simulink model "powerLoad"  (R2019b)
settings: Solver=VariableStepAuto  StartTime=0.0  StopTime=500  RelTol=1e-3
InitFcn:
  | Rho_air= 1.225;
  | C_d=0.9;
  | A_d= 0.4;
  | Static_Friction_Coefficient =0.0015;
  | Dynamic_Friction_Coefficient= 0.0015;
  | Cyclist_weight=85;
  | Vehicle_mass = 25;
  | Trailer_mass = 50;
  | g = 9.81;
  | Wheel_mass = 0.25;
  | Tire_mass = 0.25;
  | Abs = 1;
  | Bb=0.2;
  | Wheel_Radius = 0.3;
  | F_Rider = 70;
  | Wheel_Inertia=0.0225;
  | Braking_Pressure=100;
  | Crank_Length = 0.150;
  | Angle_of_crank = [0:1:360;0:1:360;]';
  | Number_of_brake_pad = 2;
  | Coefficient_of_Brake_friction = 0.9;
  | Effective_Radius_of_Disc = 0.16;
  | Outer_Radius_of_Brake = 0.18;
  | Inner_Radius_of_Brake = 0.14;
  | Disc_Mass=0;
  | Heat_capacity=0;
  | Surface_Temp=0;
  | Ambient_Temp=0;
  | Thermal_Conductivity=1;
  | 
  | Motor_torque_constant = 0.75; % NM/A
  | Kb = (51.7/(1000*2*pi/60)); %or  V/Wm (wm in rps) volt/rps
  | Jm =10.2 *10^-3; %kgm^2
  | Bm = ((Motor_torque_constant)*(17)/(1000*2*pi/60));
  | Motor_resistance =88*10^-2; %ohm
  | L = 0.36*10^-3;% H(henry)
  | alpha_Conductor =0.0040;
  | Ref_Temp = 25;
  | Alpha_Magnet = -0.0020;
  | 
  | Internal_Resistance =95*10^-3; %ohm
  | capacity =19.5 ; %Ah
  | SOC_initial = 100;
  | Polarization_Resistance = 95*10^-3;
  | Polarization_Capacitance = 1*10^-7;
undefined symbols (not defined in the file or in its folder): sigbuilder_block, V
libraries: simulink x2
(part 2 of 2)

== system powerLoad/Bike_Mechanics_subsystem/If Action Subsystem6 ==
  In1 : Inport
  Action Port : ActionPort  ActionPortLabel=else
  Gain : Gain
  Out1 : Outport
  wires:
  Gain/1 -> Out1/1
  In1/1 -> Gain/1

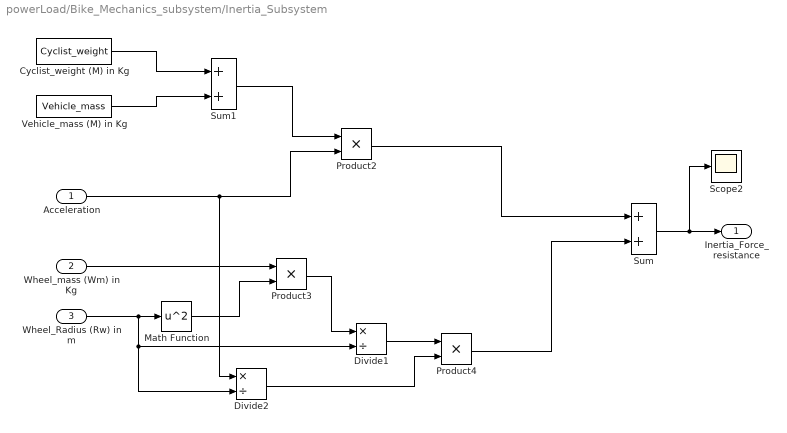
== system powerLoad/Bike_Mechanics_subsystem/Inertia_Subsystem ==
  Acceleration : Inport
  Wheel_mass (Wm) in Kg : Inport  Port=2
  Wheel_Radius (Rw) in m : Inport  Port=3
  Cyclist_weight (M) in Kg : Constant  Value=Cyclist_weight  SampleTime=-1
  Divide1 : Product  Inputs=*/
  Divide2 : Product  Inputs=*/
  Math Function : Math  Operator=square  SaturateOnIntegerOverflow=on
  Product2 : Product
  Product3 : Product
  Product4 : Product
  Scope2 : Scope
  Sum : Sum
  Sum1 : Sum
  Vehicle_mass (M) in Kg : Constant  Value=Vehicle_mass  SampleTime=-1
  Inertia_Force_resistance : Outport
  wires:
  Wheel_Radius (Rw) in m/1 -> Divide2/2, Divide1/2, Math Function/1
  Wheel_mass (Wm) in Kg/1 -> Product3/1
  Math Function/1 -> Product3/2
  Cyclist_weight (M) in Kg/1 -> Sum1/1
  Vehicle_mass (M) in Kg/1 -> Sum1/2
  Acceleration/1 -> Divide2/1, Product2/2
  Sum1/1 -> Product2/1
  Product3/1 -> Divide1/1
  Divide1/1 -> Product4/1
  Divide2/1 -> Product4/2
  Sum/1 -> Scope2/1, Inertia_Force_resistance/1
  Product2/1 -> Sum/1
  Product4/1 -> Sum/2

== system powerLoad/Bike_Mechanics_subsystem/Inertia_Subsystem1 ==
  Acceleration : Inport
  Gain : Gain
  Product2 : Product
  Scope2 : Scope
  Vehicle_mass (M) in Kg : Constant  Value=Trailer_mass  SampleTime=-1
  Trailer_force : Outport
  wires:
  Product2/1 -> Gain/1
  Vehicle_mass (M) in Kg/1 -> Product2/1
  Acceleration/1 -> Product2/2
  Gain/1 -> Scope2/1, Trailer_force/1

== system powerLoad/Bike_Mechanics_subsystem/Pedallic_torque_subsystem ==
  Torque : Inport
  Gear_ratio : Inport  Port=2
  Divide : Product  Inputs=*/
  Divide1 : Product  Inputs=*/
  Scope : Scope
  Scope1 : Scope
  Scope2 : Scope
  "Wheel_radius (Rw) " : Constant  Value=Wheel_Radius  SampleTime=-1
  Drive_Force : Outport  VectorParamsAs1DForOutWhenUnconnected=off
  wires:
  Gear_ratio/1 -> Divide1/2
  Divide1/1 -> Scope/1, Divide/1
  "Wheel_radius (Rw) "/1 -> Divide/2
  Divide/1 -> Scope2/1, Drive_Force/1
  Torque/1 -> Divide1/1, Scope1/1

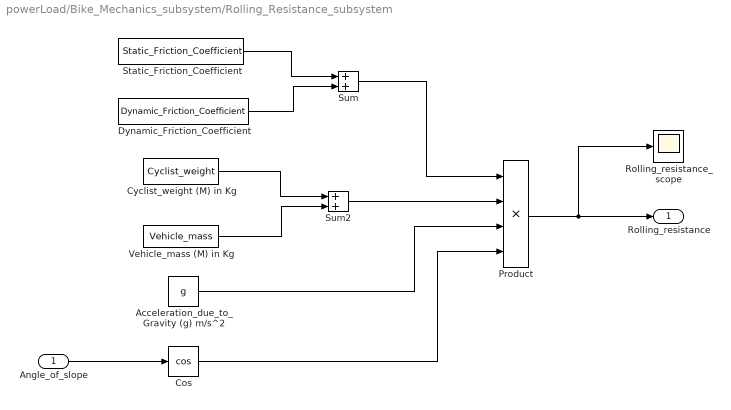
== system powerLoad/Bike_Mechanics_subsystem/Rolling_Resistance_subsystem ==
  Angle_of_slope : Inport
  Acceleration_due_to_Gravity (g) m/s^2 : Constant  Value=g  SampleTime=-1
  Cos : Trigonometry  Operator=cos
  Cyclist_weight (M) in Kg : Constant  Value=Cyclist_weight  SampleTime=-1
  Dynamic_Friction_Coefficient : Constant  Value=Dynamic_Friction_Coefficient  SampleTime=-1
  Product : Product  Inputs=4
  Rolling_resistance_scope : Scope
  Static_Friction_Coefficient : Constant  Value=Static_Friction_Coefficient  SampleTime=-1
  Sum : Sum  Inputs=+|+
  Sum2 : Sum
  Vehicle_mass (M) in Kg : Constant  Value=Vehicle_mass  SampleTime=-1
  Rolling_resistance : Outport  VectorParamsAs1DForOutWhenUnconnected=off
  wires:
  Acceleration_due_to_Gravity (g) m/s^2/1 -> Product/3
  Product/1 -> Rolling_resistance/1, Rolling_resistance_scope/1
  Cos/1 -> Product/4
  Angle_of_slope/1 -> Cos/1
  Static_Friction_Coefficient/1 -> Sum/1
  Dynamic_Friction_Coefficient/1 -> Sum/2
  Sum/1 -> Product/1
  Sum2/1 -> Product/2
  Cyclist_weight (M) in Kg/1 -> Sum2/1
  Vehicle_mass (M) in Kg/1 -> Sum2/2

== system powerLoad/Bike_Mechanics_subsystem/Subsystem2 ==
  Slope % : Inport
  Constant : Constant  Value=pi  SampleTime=-1
  Constant1 : Constant  Value=180
  Divide : Product  Inputs=*/
  Gain : Gain  Gain=1/1
  Product : Product
  Trigonometric Function : Trigonometry  Operator=atan
  alpha : Outport  VectorParamsAs1DForOutWhenUnconnected=off
  wires:
  Gain/1 -> Trigonometric Function/1
  Slope %/1 -> Gain/1
  Trigonometric Function/1 -> Product/1
  Product/1 -> alpha/1
  Constant/1 -> Divide/1
  Constant1/1 -> Divide/2
  Divide/1 -> Product/2

== system powerLoad/Controller/If Action Subsystem1 ==
  In1 : Inport
  Action Port : ActionPort  ActionPortLabel=if(u1<26)
  Gain : Gain
  Out1 : Outport
  wires:
  In1/1 -> Gain/1
  Gain/1 -> Out1/1

== system powerLoad/Controller/If Action Subsystem11 ==
  In1 : Inport
  Action Port : ActionPort  ActionPortLabel=if(u1 > 0)
  Gain : Gain  Gain=0
  Out1 : Outport
  wires:
  Gain/1 -> Out1/1
  In1/1 -> Gain/1

== system powerLoad/Controller/If Action Subsystem12 ==
  In1 : Inport
  Action Port : ActionPort  ActionPortLabel=else
  Gain : Gain
  Out1 : Outport
  wires:
  Gain/1 -> Out1/1
  In1/1 -> Gain/1

== system powerLoad/Controller/If Action Subsystem2 ==
  In1 : Inport
  Action Port : ActionPort  ActionPortLabel=if(u1 > 0)
  Gain : Gain  Gain=0
  Out1 : Outport
  wires:
  In1/1 -> Gain/1
  Gain/1 -> Out1/1

== system powerLoad/Controller/If Action Subsystem3 ==
  In1 : Inport
  Action Port : ActionPort  ActionPortLabel=else
  Gain : Gain
  Out1 : Outport
  wires:
  In1/1 -> Gain/1
  Gain/1 -> Out1/1

== system powerLoad/Controller/If Action Subsystem5 ==
  In1 : Inport
  Action Port : ActionPort  ActionPortLabel=if(u1 > 0)
  Gain : Gain  Gain=0
  Out1 : Outport
  wires:
  Gain/1 -> Out1/1
  In1/1 -> Gain/1

== system powerLoad/Controller/If Action Subsystem6 ==
  In1 : Inport
  Action Port : ActionPort  ActionPortLabel=else
  Gain : Gain
  Out1 : Outport
  wires:
  Gain/1 -> Out1/1
  In1/1 -> Gain/1

== system powerLoad/Controller/If Action Subsystem8 ==
  In1 : Inport
  Action Port : ActionPort  ActionPortLabel=else
  Gain : Gain  Gain=0
  Out1 : Outport
  wires:
  Gain/1 -> Out1/1
  In1/1 -> Gain/1

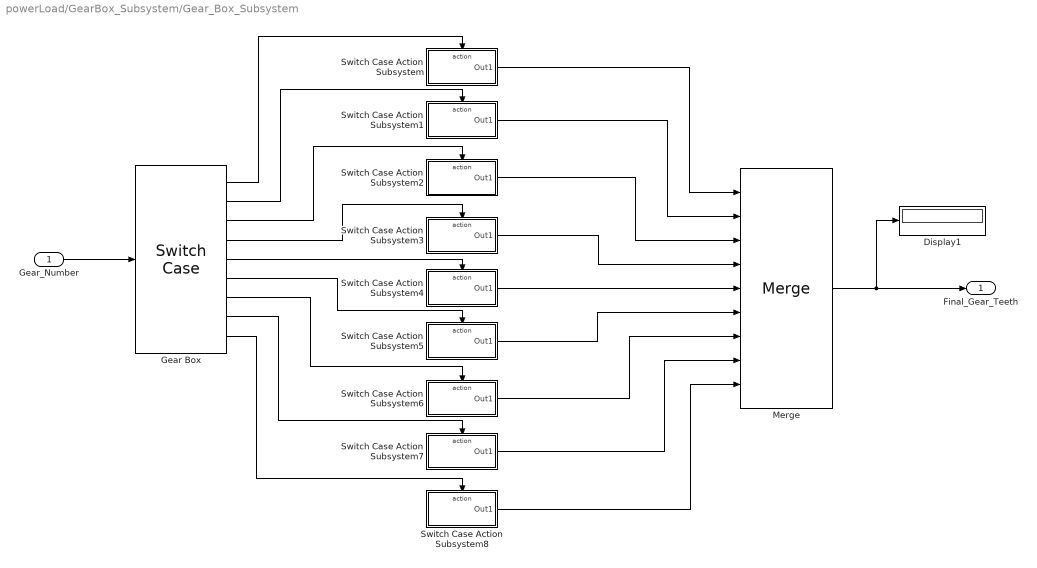
== system powerLoad/GearBox_Subsystem/Gear_Box_Subsystem ==
  Gear_Number : Inport
  Display1 : Display
  Gear Box : SwitchCase  CaseConditions={1,2,3,4,5,6,7,8,9}  ShowDefaultCase=off
  Merge : Merge  Inputs=9
  Switch Case Action Subsystem : Subsystem  TreatAsAtomicUnit=on
  Switch Case Action Subsystem1 : Subsystem  TreatAsAtomicUnit=on
  Switch Case Action Subsystem2 : Subsystem  TreatAsAtomicUnit=on
  Switch Case Action Subsystem3 : Subsystem  TreatAsAtomicUnit=on
  Switch Case Action Subsystem4 : Subsystem  TreatAsAtomicUnit=on
  Switch Case Action Subsystem5 : Subsystem  TreatAsAtomicUnit=on
  Switch Case Action Subsystem6 : Subsystem  TreatAsAtomicUnit=on
  Switch Case Action Subsystem7 : Subsystem  TreatAsAtomicUnit=on
  Switch Case Action Subsystem8 : Subsystem  TreatAsAtomicUnit=on
  Final_Gear_Teeth : Outport  VectorParamsAs1DForOutWhenUnconnected=off
  wires:
  Gear Box/5 -> Switch Case Action Subsystem4/Action
  Gear Box/2 -> Switch Case Action Subsystem1/Action
  Gear Box/4 -> Switch Case Action Subsystem3/Action
  Gear Box/9 -> Switch Case Action Subsystem8/Action
  Gear Box/7 -> Switch Case Action Subsystem6/Action
  Gear Box/6 -> Switch Case Action Subsystem5/Action
  Gear Box/3 -> Switch Case Action Subsystem2/Action
  Gear Box/1 -> Switch Case Action Subsystem/Action
  Merge/1 -> Display1/1, Final_Gear_Teeth/1
  Gear Box/8 -> Switch Case Action Subsystem7/Action
  Gear_Number/1 -> Gear Box/1
  Switch Case Action Subsystem8/1(Out1) -> Merge/9
  Switch Case Action Subsystem7/1(Out1) -> Merge/8
  Switch Case Action Subsystem6/1(Out1) -> Merge/7
  Switch Case Action Subsystem5/1(Out1) -> Merge/6
  Switch Case Action Subsystem4/1(Out1) -> Merge/5
  Switch Case Action Subsystem3/1(Out1) -> Merge/4
  Switch Case Action Subsystem2/1(Out1) -> Merge/3
  Switch Case Action Subsystem1/1(Out1) -> Merge/2
  Switch Case Action Subsystem/1(Out1) -> Merge/1

== system powerLoad/Motor_Subsystem/Magnetic_Flux_density_subsystem ==
  Ambient_temp_T : Inport
  Motor_torque_constant_at_Temp_T0 : Inport  Port=2
  Constant : Constant
  Product : Product
  Product1 : Product
  Reference_temp_T0 : Constant  Value=Ref_Temp
  Sum1 : Sum  Inputs=+-
  Sum2 : Sum
  Temperature_Coefficient : Constant  Value=Alpha_Magnet
  Motor_Torque_Constant_at_Temp_T : Outport  VectorParamsAs1DForOutWhenUnconnected=off
  wires:
  Motor_torque_constant_at_Temp_T0/1 -> Product1/1
  Product1/1 -> Motor_Torque_Constant_at_Temp_T/1
  Product/1 -> Sum2/2
  Constant/1 -> Sum2/1
  Sum2/1 -> Product1/2
  Temperature_Coefficient/1 -> Product/1
  Ambient_temp_T/1 -> Sum1/1
  Reference_temp_T0/1 -> Sum1/2
  Sum1/1 -> Product/2

== system powerLoad/Motor_Subsystem/Winding_resistance_Subsystem ==
  Resistance_at_Temp_T0 : Inport
  Ambient_temp_T : Inport  Port=2
  Constant : Constant
  Product : Product
  Product1 : Product
  Reference_temp_T0 : Constant  Value=Ref_Temp
  Resistance_Temperature_Coefficient : Constant  Value=alpha_Conductor
  Sum1 : Sum  Inputs=+-
  Sum2 : Sum
  Resistance_at_Temp_T : Outport  VectorParamsAs1DForOutWhenUnconnected=off
  wires:
  Sum1/1 -> Product/2
  Reference_temp_T0/1 -> Sum1/2
  Ambient_temp_T/1 -> Sum1/1
  Resistance_Temperature_Coefficient/1 -> Product/1
  Sum2/1 -> Product1/2
  Constant/1 -> Sum2/1
  Product/1 -> Sum2/2
  Product1/1 -> Resistance_at_Temp_T/1
  Resistance_at_Temp_T0/1 -> Product1/1

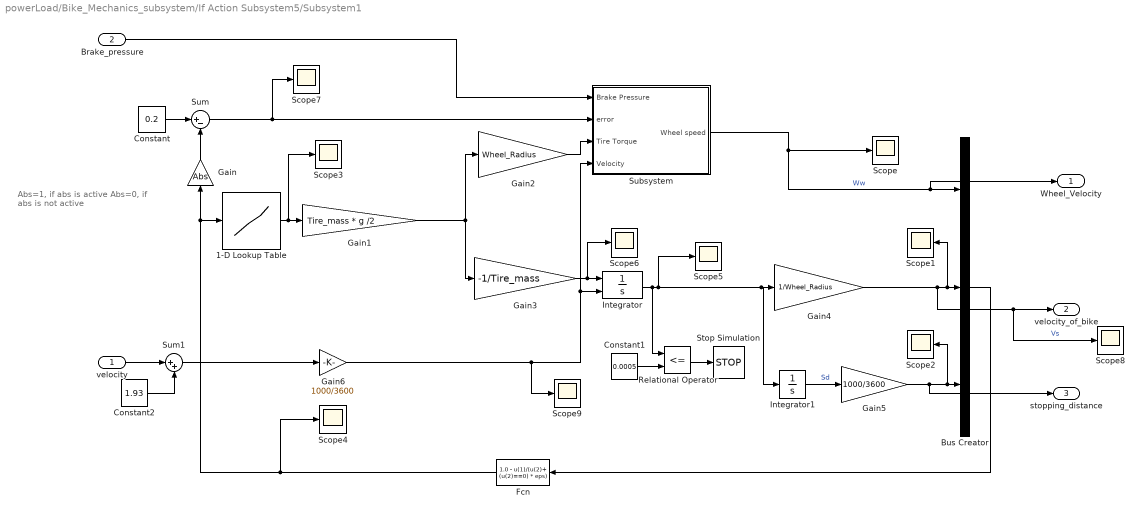
== system powerLoad/Bike_Mechanics_subsystem/If Action Subsystem5/Subsystem1 ==
  note: Abs=1, if abs is active
      | Abs=0, if abs is not active
  velocity : Inport
  Brake_pressure : Inport  Port=2
  1-D Lookup Table : Lookup_n-D  NumberOfTableDimensions=1  BreakpointsForDimension1="[0\t0.0500000000000000\t0.100000000000000\t0.150000000000000\t0.200000000000000\t0.250000000000000\t0.300000000000000\t0.350000000000000\t0.400000000000000\t0.450000000000000\t0.500000000000000\t0.550000000000000\t0.600000000000000\t0.650000000000000\t0.700000000000000\t0.750000000000000\t0.800000000000000\t0.850000000000000\t0.900000000000000\t0.950000000000000\t1]"  Table="[0\t0.400000000000000\t0.800000000000000\t0.970000000000000\t1\t0.980000000000000\t0.960000000000000\t0.940000000000000\t0.920000000000000\t0.900000000000000\t0.880000000000000\t0.855000000000000\t0.830000000000000\t0.810000000000000\t0.790000000000000\t0.770000000000000\t0.750000000000000\t0.730000000000000\t0.720000000000000\t0.710000000000000\t0.700000000000000]"  InternalRulePriority=Speed  RndMeth=Simplest  InputSameDT=on
  Bus Creator : BusCreator  Inputs=3
  Constant : Constant  Value=0.2
  Constant1 : Constant  Value=0.0005
  Constant2 : Constant  Value=1.93
  Fcn : Fcn  Expr=1.0 - u(1)/(u(2)+ (u(2)==0) * eps)
  Gain : Gain  Gain=Abs
  Gain1 : Gain  Gain=Tire_mass * g /2
  Gain2 : Gain  Gain=Wheel_Radius
  Gain3 : Gain  Gain=-1/Tire_mass
  Gain4 : Gain  Gain=1/Wheel_Radius
  Gain5 : Gain  Gain=1000/3600
  Gain6 : Gain  Gain=1000/3600
  Integrator : Integrator  InitialConditionSource=external  InitialCondition=V  LimitOutput=on  UpperSaturationLimit=1000  LowerSaturationLimit=0  ZeroCross=off
  Integrator1 : Integrator
  Relational Operator : RelationalOperator  Operator=<=  OutDataTypeStr=boolean  RndMeth=Simplest
  Scope{,1..9} (10 alike) : Scope
  Stop Simulation : Stop
  Subsystem : Subsystem
  Sum : Sum  Inputs=|+-
  Sum1 : Sum  Inputs=|++
  Wheel_Velocity : Outport
  velocity_of_bike : Outport  Port=2
  stopping_distance : Outport  Port=3
  wires:
  Subsystem/1("Wheel speed ") -> Scope/1, Wheel_Velocity/1, Bus Creator/1  "Ww"
  Integrator1/1 -> Gain5/1  "Sd"
  Sum/1 -> Subsystem/2("error "), Scope7/1
  Gain1/1 -> Gain3/1, Gain2/1
  Gain2/1 -> Subsystem/3(Tire Torque)
  Gain/1 -> Sum/2
  1-D Lookup Table/1 -> Scope3/1, Gain1/1
  Gain3/1 -> Scope6/1, Integrator/1
  Constant/1 -> Sum/1
  Gain4/1 -> Scope1/1, Bus Creator/2, Scope8/1, velocity_of_bike/1  "Vs"
  Fcn/1 -> Scope4/1, 1-D Lookup Table/1, Gain/1
  Bus Creator/1 -> Fcn/1
  Constant1/1 -> Relational Operator/2
  Relational Operator/1 -> Stop Simulation/1
  Integrator/1 -> Integrator1/1, Gain4/1, Scope5/1, Relational Operator/1
  Gain5/1 -> stopping_distance/1, Scope2/1, Bus Creator/3
  Gain6/1 -> Scope9/1, Subsystem/4(Velocity), Integrator/2
  Brake_pressure/1 -> Subsystem/1(Brake Pressure)
  velocity/1 -> Sum1/1
  Constant2/1 -> Sum1/2
  Sum1/1 -> Gain6/1

== system powerLoad/GearBox_Subsystem/Gear_Box_Subsystem/Switch Case Action Subsystem ==
  Action Port : ActionPort  ActionPortLabel=case [ 1 ]:
  Constant : Constant  Value=34
  Out1 : Outport  VectorParamsAs1DForOutWhenUnconnected=off
  wires:
  Constant/1 -> Out1/1

== system powerLoad/GearBox_Subsystem/Gear_Box_Subsystem/Switch Case Action Subsystem1 ==
  Action Port : ActionPort  ActionPortLabel=case [ 2 ]:
  Constant : Constant  Value=30
  Out1 : Outport  VectorParamsAs1DForOutWhenUnconnected=off
  wires:
  Constant/1 -> Out1/1

== system powerLoad/GearBox_Subsystem/Gear_Box_Subsystem/Switch Case Action Subsystem2 ==
  Action Port : ActionPort  ActionPortLabel=case [ 3 ]:
  Constant : Constant  Value=26
  Out1 : Outport  VectorParamsAs1DForOutWhenUnconnected=off
  wires:
  Constant/1 -> Out1/1

== system powerLoad/GearBox_Subsystem/Gear_Box_Subsystem/Switch Case Action Subsystem3 ==
  Action Port : ActionPort  ActionPortLabel=case [ 4 ]:
  Constant : Constant  Value=23
  Out1 : Outport  VectorParamsAs1DForOutWhenUnconnected=off
  wires:
  Constant/1 -> Out1/1

== system powerLoad/GearBox_Subsystem/Gear_Box_Subsystem/Switch Case Action Subsystem4 ==
  Action Port : ActionPort  ActionPortLabel=case [ 5 ]:
  Constant : Constant  Value=20
  Out1 : Outport  VectorParamsAs1DForOutWhenUnconnected=off
  wires:
  Constant/1 -> Out1/1

== system powerLoad/GearBox_Subsystem/Gear_Box_Subsystem/Switch Case Action Subsystem5 ==
  Action Port : ActionPort  ActionPortLabel=case [ 6 ]:
  Constant : Constant  Value=17
  Out1 : Outport  VectorParamsAs1DForOutWhenUnconnected=off
  wires:
  Constant/1 -> Out1/1

== system powerLoad/GearBox_Subsystem/Gear_Box_Subsystem/Switch Case Action Subsystem6 ==
  Action Port : ActionPort  ActionPortLabel=case [ 7 ]:
  Constant : Constant  Value=15
  Out1 : Outport  VectorParamsAs1DForOutWhenUnconnected=off
  wires:
  Constant/1 -> Out1/1

== system powerLoad/GearBox_Subsystem/Gear_Box_Subsystem/Switch Case Action Subsystem7 ==
  Action Port : ActionPort  ActionPortLabel=case [ 8 ]:
  Constant : Constant  Value=13
  Out1 : Outport  VectorParamsAs1DForOutWhenUnconnected=off
  wires:
  Constant/1 -> Out1/1

== system powerLoad/GearBox_Subsystem/Gear_Box_Subsystem/Switch Case Action Subsystem8 ==
  Action Port : ActionPort  ActionPortLabel=case [ 9 ]:
  Constant : Constant  Value=11
  Out1 : Outport  VectorParamsAs1DForOutWhenUnconnected=off
  wires:
  Constant/1 -> Out1/1

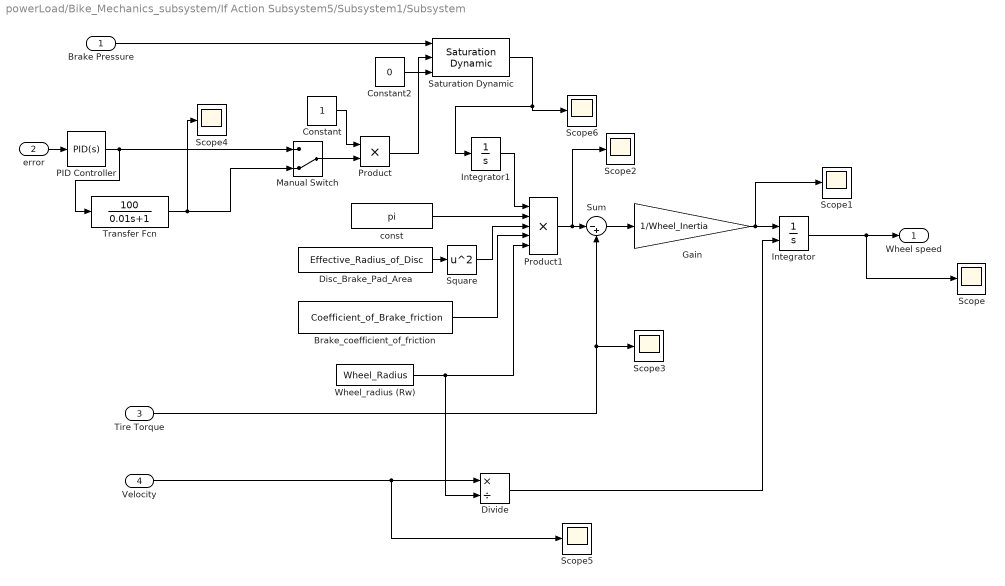
== system powerLoad/Bike_Mechanics_subsystem/If Action Subsystem5/Subsystem1/Subsystem ==
  Brake Pressure : Inport
  "error " : Inport  Port=2
  Tire Torque : Inport  Port=3
  Velocity : Inport  Port=4
  Brake_coefficient_of_friction : Constant  Value=Coefficient_of_Brake_friction
  Constant : Constant
  Constant2 : Constant  Value=0
  Disc_Brake_Pad_Area : Constant  Value=Effective_Radius_of_Disc
  Divide : Product  Inputs=*/
  Gain : Gain  Gain=1/Wheel_Inertia
  Integrator : Integrator  InitialConditionSource=external  InitialCondition=V/Wheel_Radius  LimitOutput=on  UpperSaturationLimit=1000  LowerSaturationLimit=0
  Integrator1 : Integrator  UpperSaturationLimit=Braking_Pressure
  Manual Switch : ManualSwitch  CurrentSetting=0
  PID Controller : simulink/Continuous/PID Controller  Controller=PID  Form=Parallel  TimeDomain=Continuous-time  SampleTime=-1  IntegratorMethod=Forward Euler  FilterMethod=Forward Euler  ControllerParametersSource=internal  P=22  I=4  D=0.4  UseFilter=on  N=100  TunerSelectOption=Transfer Function Based (PID Tuner App)  InitialConditionSource=internal  InitialConditionForIntegrator=0  InitialConditionForFilter=0  DifferentiatorICPrevScaledInput=0  ExternalReset=none  TrackingMode=off  Kt=1  LimitOutput=off  UpperSaturationLimit=inf  LowerSaturationLimit=-inf  LinearizeAsGain=on  AntiWindupMode=none  Kb=1  POutMin=[]  POutMax=[]  IOutMin=[]  IOutMax=[]  DOutMin=[]  DOutMax=[]  NOutMin=[]  NOutMax=[]  SumOutMin=[]  SumOutMax=[]  SaturationOutMin=[]  SaturationOutMax=[]  PParamMin=[]  PParamMax=[]  IParamMin=[]  IParamMax=[]  DParamMin=[]  DParamMax=[]  NParamMin=[]  NParamMax=[]  KbParamMin=[]  KbParamMax=[]  KtParamMin=[]  KtParamMax=[]  KbOutMin=[]  KbOutMax=[]  KtOutMin=[]  KtOutMax=[]  IntegratorOutMin=[]  IntegratorOutMax=[]  FilterOutMin=[]  FilterOutMax=[]  SumI1OutMin=[]  SumI1OutMax=[]  SumI2OutMin=[]  SumI2OutMax=[]  SumI3OutMin=[]  SumI3OutMax=[]  SumI4OutMin=[]  SumI4OutMax=[]  SumDOutMin=[]  SumDOutMax=[]  DifferentiatorOutMin=[]  DifferentiatorOutMax=[]  FilterDiffOutCoefMin=[]  FilterDiffOutCoefMax=[]  ReciprocalOutMin=[]  ReciprocalOutMax=[]  SumDenOutMin=[]  SumDenOutMax=[]  SumNumOutMin=[]  SumNumOutMax=[]  DivideOutMin=[]  DivideOutMax=[]  IntegratorContinuousStateAttributes=''  IntegratorStateMustResolveToSignalObject=off  IntegratorRTWStateStorageClass=Auto  FilterContinuousStateAttributes=''  FilterStateMustResolveToSignalObject=off  FilterRTWStateStorageClass=Auto  ParallelPVariant=InternalParameters  IdealPVariant=Disabled  IVariant=InternalParameters  DVariant=InternalParameters  IntegratorVariant=Continuous  SatVariant=Disabled  AWVariant=Passthrough  PCopyVariant=Disabled  TRVariant=Disabled  FdbkBlocksVariant=Forward  IdealPFdbkVariant=Disabled  SatFdbkVariant=Disabled  DerivativeFilterVariant=ContFilter  NVariant=InternalParameters  NCopyVariant=Disabled  FilterICVariant=InternalICsFilter  IntegratorICVariant=InternalICs  ExternalResetVariant=Disabled  TRSumVariant=Passthrough  SumFdbkVariant=Disabled  SumVariant=Sum_PID
  Product : Product
  Product1 : Product  Inputs=5
  Saturation Dynamic : simulink/Discontinuities/Saturation Dynamic  OutMin=[]  OutMax=[]  OutDataTypeStr=Inherit: Same as second input  OutDataType=fixdt(1, 16)  OutScaling=2^-10  DoSatur=off
  Scope{,1..6} (7 alike) : Scope
  Square : Math  Operator=square  SaturateOnIntegerOverflow=on
  Sum : Sum  Inputs=|-+
  Transfer Fcn : TransferFcn  Numerator=[100]  Denominator=[0.01 1]
  "Wheel_radius (Rw) " : Constant  Value=Wheel_Radius
  "const " : Constant  Value=pi
  "Wheel speed " : Outport
  wires:
  "error "/1 -> PID Controller/1
  Constant/1 -> Product/1
  "const "/1 -> Product1/2
  Disc_Brake_Pad_Area/1 -> Square/1
  Square/1 -> Product1/3
  Brake_coefficient_of_friction/1 -> Product1/4
  Product1/1 -> Scope2/1, Sum/1
  Tire Torque/1 -> Scope3/1, Sum/2
  Sum/1 -> Gain/1
  Gain/1 -> Scope1/1, Integrator/1
  Manual Switch/1 -> Product/2
  PID Controller/1 -> Transfer Fcn/1, Manual Switch/1
  Integrator1/1 -> Product1/1
  Velocity/1 -> Scope5/1, Divide/1
  Divide/1 -> Integrator/2
  "Wheel_radius (Rw) "/1 -> Divide/2, Product1/5
  Integrator/1 -> "Wheel speed "/1, Scope/1
  Transfer Fcn/1 -> Scope4/1, Manual Switch/2
  Constant2/1 -> Saturation Dynamic/3
  Product/1 -> Saturation Dynamic/2
  Saturation Dynamic/1 -> Scope6/1, Integrator1/1
  Brake Pressure/1 -> Saturation Dynamic/1
